simulink model "Final_Leg_Walk_V1"  (R2025b)
settings: Solver=VariableStepAuto  StartTime=0.0  StopTime=150  RelTol=0.01  AbsTol=0.01  EnableMultiTasking=on
undefined symbols (not defined in the file): X, Y, Z
libraries: sm_lib x54, nesl_utility x13
(part 3 of 3)

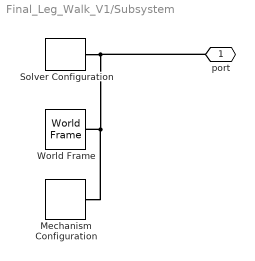
== system Final_Leg_Walk_V1/Subsystem ==
  Mechanism Configuration : sm_lib/Utilities/Mechanism Configuration  UniformGravity=Constant  GravityVector=[0 0 -9.80665]  GravityVectorUnits=m/s^2  LinearizationDelta=0.001  JointModeTransitionNonlinearIterations=2
  Solver Configuration : nesl_utility/Solver Configuration  PhysicalDomain=network_engine_domain  SubClassName=solver  LeftPortType=input  RightPortType=generic  Tones=[]  Harmonics=[]  SimulateNoise=off  Profile=off  UseLocalSampling=off  EnableSwitchedLinearOptims=on  FrequencyDomain=off  UseCCode=off  RelTol=0.001  AbsTol=1e-06  MinStep=1e-09  ToWorkspace=off  RevertToSquareIcSolve=off  NumHomotopyIterations=100  PhasorMode=off  PhasorModeNumHarmonics=1  ConsistencySolver=NEWTON_XTOL_AFTER_FTOL  IndexReductionMethod=DerivativeReplacement  DoDC=off  ResidualTolerance=1e-09  ConsistencyTolSource=GLOBAL  ConsistencyAbsTol=0.001  ConsistencyRelTol=0.001  ConsistencyTolFactor=0.001  UseLocalSolver=off  LocalSolverChoice=NE_BACKWARD_EULER_ADVANCER  ResolveIndetEquations=on  FunctionEvalNumThread=1  LocalSolverSampleTime=0.001  DoFixedCost=off  MaxNonlinIter=3  MaxModeIter=2  ComputeImpulses=off  ImpulseIterations=2  LinearAlgebra=Sparse  LinearAlgebraNumThread=0  EquationFormulation=NE_TIME_EF  DelaysMemoryBudget=1024  AutomaticFiltering=on  FilteringTimeConstant=0.001  PartitionStorageMethod=AS_NEEDED  PartitionMemoryBudget=1024  PartitionMethod=FAST  MultibodyUseLocalSolver=off  MultibodyLocalSolverChoice=ODE1  MultibodyLocalSolverSampleTime=0.001
  World Frame : sm_lib/Frames and Transforms/World Frame
  port : PMIOPort  Side=Right
  connections:
  Solver Configuration/RConn1 -- port/RConn1 -- Mechanism Configuration/RConn1 -- World Frame/RConn1

== matlab function Final_Leg_Walk_V1/RR/MATLAB Function3 ==
  data: t input; q_roll output; leg_id input; q_hip output; q_knee output
function [q_roll, q_hip, q_knee] = motion_walker_v8_extended(t, leg_id)
    % (small stepping + large backward stroke) extended to a complete
    % four-leg cycle
    % Sequence: right front (0) -> left rear (2) -> left front (1) -> right rear (3)
    
    % ================= settings =================
    T_start = 2.0;
    if t < T_start
        q_roll = 0; q_hip = 0; q_knee = 0;
        return;
    end
    t_run = t - T_start;
    
    % [1] Lean(roll) amplitude
    ang_lean = deg2rad(3); 
    
    % [2] Step amplitude (negative value moves forward)
    ang_step = deg2rad(-10); 
    
    % [3] Propulsion amplitude (positive value moves backword)
    ang_push = deg2rad(10);
    
    % [4] Leg lift amplitude
    ang_lift = deg2rad(-12); 
    
    % Period: 4 legs x (2s preparation + 2s action)=16s
    T_cycle = 16.0; 
    tau = mod(t_run, T_cycle);
    
    smooth_move = @(x) (1 - cos(x*pi))/2; 
    lift_arch   = @(x) sin(x*pi);         

    % ================= Logic =================
    q_roll = 0; q_hip = 0; q_knee = 0;
    
    % ---------------------------------------------------------
    % Phase A: Right Front, Leg 0 [0-4s]
    % ---------------------------------------------------------
    if tau < 2.0
        % [Preparation] Shift the center of mass to the left (0 -> -5)
        s = smooth_move(tau/2.0);
        q_roll = s * (-ang_lean);

        
    elseif tau < 4.0
        % [Action] Lift the right front leg
        local_t = (tau - 2.0)/2.0;
        s = smooth_move(local_t);
        q_roll = -ang_lean; % maintain left lean
        
        if leg_id == 0
            % === Main leg: right front leg ===
            q_knee = lift_arch(local_t) * ang_lift;
            q_hip = s * ang_step; 
        else
            % === Supporting legs: other legs ===
            q_knee = 0; 
            q_hip = s * ang_push; % continue backward stroke
        end

    % ---------------------------------------------------------
    % Phase B: Left Rear, Leg 2 [4-8s]
    % ---------------------------------------------------------
    elseif tau < 6.0
        % [Preparation] Shift the center of mass to the right (-5 -> +5)
        local_t = (tau - 4.0)/2.0;
        s = smooth_move(local_t);
        q_roll = -ang_lean + s * (2 * ang_lean);
        
        % Keep the leg that just stepped forward in place; the others keep
        % stroking backward
        if leg_id == 0; q_hip = ang_step; else; q_hip = ang_push; end
        
    elseif tau < 8.0
        % [Action] Lift the left rear leg
        local_t = (tau - 6.0)/2.0;
        s = smooth_move(local_t);
        q_roll = ang_lean; % Maintain right lean
        
        if leg_id == 2
            % === Main leg: left rear leg ===
            q_knee = lift_arch(local_t) * ang_lift;
            q_hip = ang_push + s * (ang_step - ang_push); % Step forward
        else
            % === Supporting legs: other legs ===
            q_knee = 0;
            % Right front leg(0) stays forward, other legs stay backward
            if leg_id == 0; q_hip = ang_step; else; q_hip = ang_push; end
        end

    % ---------------------------------------------------------
    % Phase C: Left Front, Leg 1 [8-12s]
    % ---------------------------------------------------------
    elseif tau < 10.0
         % [Preparation] Keep the center of mass on the right side (no movement)
         % Because the previous motion was the left rear leg (COM on the right),
         % and now the left front leg moves, the COM must remain on the right
        q_roll = ang_lean; 
        
        if leg_id == 0 || leg_id == 2; q_hip = ang_step; else; q_hip = ang_push; end
        
    elseif tau < 12.0
        % [Action] Lift the left front leg
        local_t = (tau - 10.0)/2.0;
        s = smooth_move(local_t);
        q_roll = ang_lean; % Maintain right lean
        
        if leg_id == 1
            % === Main leg: left front leg ===
            q_knee = lift_arch(local_t) * ang_lift;
            q_hip = ang_push + s * (ang_step - ang_push);
        else
            q_knee = 0;
            if leg_id == 0 || leg_id == 2; q_hip = ang_step; else; q_hip = ang_push; end
        end

    % ---------------------------------------------------------
    % Phase D: Right Rear, Leg 3 [12-16s]
    % ---------------------------------------------------------
    elseif tau < 14.0
        % [Preparation] Shift the center of mass from right back to the left (+5 -> -5)
        local_t = (tau - 12.0)/2.0;
        s = smooth_move(local_t);
        q_roll = ang_lean + s * (-2 * ang_lean);
        
        if leg_id == 3; q_hip = ang_push; else; q_hip = ang_step; end
        
    else
        % [Action] Lift the right rear leg
        local_t = (tau - 14.0)/2.0;
        s = smooth_move(local_t);
        q_roll = -ang_lean * (1 - s); % Left lean gradually returns to neutral
        target_pos = 0; 
        if leg_id == 3
            % === Main leg: right rear leg ===
            q_knee = lift_arch(local_t) * ang_lift;
            q_hip = ang_push + s * (target_pos - ang_push);
        else
            q_knee = 0;
            % All other legs return to neutral
            q_hip = ang_step + s * (target_pos - ang_step);
            
        end
    end
end

== matlab function Final_Leg_Walk_V1/FL/MATLAB Function3 ==
  data: t input; q_roll output; leg_id input; q_hip output; q_knee output
function [q_roll, q_hip, q_knee] = motion_walker_v8_extended(t, leg_id)
    % (small stepping + large backward stroke) extended to a complete
    % four-leg cycle
    % Sequence: right front (0) -> left rear (2) -> left front (1) -> right rear (3)
    
    % ================= settings =================
    T_start = 2.0;
    if t < T_start
        q_roll = 0; q_hip = 0; q_knee = 0;
        return;
    end
    t_run = t - T_start;
    
    % [1] Lean(roll) amplitude
    ang_lean = deg2rad(3); 
    
    % [2] Step amplitude (negative value moves forward)
    ang_step = deg2rad(-10); 
    
    % [3] Propulsion amplitude (positive value moves backword)
    ang_push = deg2rad(10);
    
    % [4] Leg lift amplitude
    ang_lift = deg2rad(-12); 
    
    % Period: 4 legs x (2s preparation + 2s action)=16s
    T_cycle = 16.0; 
    tau = mod(t_run, T_cycle);
    
    smooth_move = @(x) (1 - cos(x*pi))/2; 
    lift_arch   = @(x) sin(x*pi);         

    % ================= Logic =================
    q_roll = 0; q_hip = 0; q_knee = 0;
    
    % ---------------------------------------------------------
    % Phase A: Right Front, Leg 0 [0-4s]
    % ---------------------------------------------------------
    if tau < 2.0
        % [Preparation] Shift the center of mass to the left (0 -> -5)
        s = smooth_move(tau/2.0);
        q_roll = s * (-ang_lean);

        
    elseif tau < 4.0
        % [Action] Lift the right front leg
        local_t = (tau - 2.0)/2.0;
        s = smooth_move(local_t);
        q_roll = -ang_lean; % maintain left lean
        
        if leg_id == 0
            % === Main leg: right front leg ===
            q_knee = lift_arch(local_t) * ang_lift;
            q_hip = s * ang_step; 
        else
            % === Supporting legs: other legs ===
            q_knee = 0; 
            q_hip = s * ang_push; % continue backward stroke
        end

    % ---------------------------------------------------------
    % Phase B: Left Rear, Leg 2 [4-8s]
    % ---------------------------------------------------------
    elseif tau < 6.0
        % [Preparation] Shift the center of mass to the right (-5 -> +5)
        local_t = (tau - 4.0)/2.0;
        s = smooth_move(local_t);
        q_roll = -ang_lean + s * (2 * ang_lean);
        
        % Keep the leg that just stepped forward in place; the others keep
        % stroking backward
        if leg_id == 0; q_hip = ang_step; else; q_hip = ang_push; end
        
    elseif tau < 8.0
        % [Action] Lift the left rear leg
        local_t = (tau - 6.0)/2.0;
        s = smooth_move(local_t);
        q_roll = ang_lean; % Maintain right lean
        
        if leg_id == 2
            % === Main leg: left rear leg ===
            q_knee = lift_arch(local_t) * ang_lift;
            q_hip = ang_push + s * (ang_step - ang_push); % Step forward
        else
            % === Supporting legs: other legs ===
            q_knee = 0;
            % Right front leg(0) stays forward, other legs stay backward
            if leg_id == 0; q_hip = ang_step; else; q_hip = ang_push; end
        end

    % ---------------------------------------------------------
    % Phase C: Left Front, Leg 1 [8-12s]
    % ---------------------------------------------------------
    elseif tau < 10.0
         % [Preparation] Keep the center of mass on the right side (no movement)
         % Because the previous motion was the left rear leg (COM on the right),
         % and now the left front leg moves, the COM must remain on the right
        q_roll = ang_lean; 
        
        if leg_id == 0 || leg_id == 2; q_hip = ang_step; else; q_hip = ang_push; end
        
    elseif tau < 12.0
        % [Action] Lift the left front leg
        local_t = (tau - 10.0)/2.0;
        s = smooth_move(local_t);
        q_roll = ang_lean; % Maintain right lean
        
        if leg_id == 1
            % === Main leg: left front leg ===
            q_knee = lift_arch(local_t) * ang_lift;
            q_hip = ang_push + s * (ang_step - ang_push);
        else
            q_knee = 0;
            if leg_id == 0 || leg_id == 2; q_hip = ang_step; else; q_hip = ang_push; end
        end

    % ---------------------------------------------------------
    % Phase D: Right Rear, Leg 3 [12-16s]
    % ---------------------------------------------------------
    elseif tau < 14.0
        % [Preparation] Shift the center of mass from right back to the left (+5 -> -5)
        local_t = (tau - 12.0)/2.0;
        s = smooth_move(local_t);
        q_roll = ang_lean + s * (-2 * ang_lean);
        
        if leg_id == 3; q_hip = ang_push; else; q_hip = ang_step; end
        
    else
        % [Action] Lift the right rear leg
        local_t = (tau - 14.0)/2.0;
        s = smooth_move(local_t);
        q_roll = -ang_lean * (1 - s); % Left lean gradually returns to neutral
        target_pos = 0; 
        if leg_id == 3
            % === Main leg: right rear leg ===
            q_knee = lift_arch(local_t) * ang_lift;
            q_hip = ang_push + s * (target_pos - ang_push);
        else
            q_knee = 0;
            % All other legs return to neutral
            q_hip = ang_step + s * (target_pos - ang_step);
            
        end
    end
end

== matlab function Final_Leg_Walk_V1/FR/MATLAB Function3 ==
  data: t input; q_roll output; leg_id input; q_hip output; q_knee output
function [q_roll, q_hip, q_knee] = motion_walker_v8_extended(t, leg_id)
    % (small stepping + large backward stroke) extended to a complete
    % four-leg cycle
    % Sequence: right front (0) -> left rear (2) -> left front (1) -> right rear (3)
    
    % ================= settings =================
    T_start = 2.0;
    if t < T_start
        q_roll = 0; q_hip = 0; q_knee = 0;
        return;
    end
    t_run = t - T_start;
    
    % [1] Lean(roll) amplitude
    ang_lean = deg2rad(3); 
    
    % [2] Step amplitude (negative value moves forward)
    ang_step = deg2rad(-10); 
    
    % [3] Propulsion amplitude (positive value moves backword)
    ang_push = deg2rad(10);
    
    % [4] Leg lift amplitude
    ang_lift = deg2rad(-12); 
    
    % Period: 4 legs x (2s preparation + 2s action)=16s
    T_cycle = 16.0; 
    tau = mod(t_run, T_cycle);
    
    smooth_move = @(x) (1 - cos(x*pi))/2; 
    lift_arch   = @(x) sin(x*pi);         

    % ================= Logic =================
    q_roll = 0; q_hip = 0; q_knee = 0;
    
    % ---------------------------------------------------------
    % Phase A: Right Front, Leg 0 [0-4s]
    % ---------------------------------------------------------
    if tau < 2.0
        % [Preparation] Shift the center of mass to the left (0 -> -5)
        s = smooth_move(tau/2.0);
        q_roll = s * (-ang_lean);

        
    elseif tau < 4.0
        % [Action] Lift the right front leg
        local_t = (tau - 2.0)/2.0;
        s = smooth_move(local_t);
        q_roll = -ang_lean; % maintain left lean
        
        if leg_id == 0
            % === Main leg: right front leg ===
            q_knee = lift_arch(local_t) * ang_lift;
            q_hip = s * ang_step; 
        else
            % === Supporting legs: other legs ===
            q_knee = 0; 
            q_hip = s * ang_push; % continue backward stroke
        end

    % ---------------------------------------------------------
    % Phase B: Left Rear, Leg 2 [4-8s]
    % ---------------------------------------------------------
    elseif tau < 6.0
        % [Preparation] Shift the center of mass to the right (-5 -> +5)
        local_t = (tau - 4.0)/2.0;
        s = smooth_move(local_t);
        q_roll = -ang_lean + s * (2 * ang_lean);
        
        % Keep the leg that just stepped forward in place; the others keep
        % stroking backward
        if leg_id == 0; q_hip = ang_step; else; q_hip = ang_push; end
        
    elseif tau < 8.0
        % [Action] Lift the left rear leg
        local_t = (tau - 6.0)/2.0;
        s = smooth_move(local_t);
        q_roll = ang_lean; % Maintain right lean
        
        if leg_id == 2
            % === Main leg: left rear leg ===
            q_knee = lift_arch(local_t) * ang_lift;
            q_hip = ang_push + s * (ang_step - ang_push); % Step forward
        else
            % === Supporting legs: other legs ===
            q_knee = 0;
            % Right front leg(0) stays forward, other legs stay backward
            if leg_id == 0; q_hip = ang_step; else; q_hip = ang_push; end
        end

    % ---------------------------------------------------------
    % Phase C: Left Front, Leg 1 [8-12s]
    % ---------------------------------------------------------
    elseif tau < 10.0
         % [Preparation] Keep the center of mass on the right side (no movement)
         % Because the previous motion was the left rear leg (COM on the right),
         % and now the left front leg moves, the COM must remain on the right
        q_roll = ang_lean; 
        
        if leg_id == 0 || leg_id == 2; q_hip = ang_step; else; q_hip = ang_push; end
        
    elseif tau < 12.0
        % [Action] Lift the left front leg
        local_t = (tau - 10.0)/2.0;
        s = smooth_move(local_t);
        q_roll = ang_lean; % Maintain right lean
        
        if leg_id == 1
            % === Main leg: left front leg ===
            q_knee = lift_arch(local_t) * ang_lift;
            q_hip = ang_push + s * (ang_step - ang_push);
        else
            q_knee = 0;
            if leg_id == 0 || leg_id == 2; q_hip = ang_step; else; q_hip = ang_push; end
        end

    % ---------------------------------------------------------
    % Phase D: Right Rear, Leg 3 [12-16s]
    % ---------------------------------------------------------
    elseif tau < 14.0
        % [Preparation] Shift the center of mass from right back to the left (+5 -> -5)
        local_t = (tau - 12.0)/2.0;
        s = smooth_move(local_t);
        q_roll = ang_lean + s * (-2 * ang_lean);
        
        if leg_id == 3; q_hip = ang_push; else; q_hip = ang_step; end
        
    else
        % [Action] Lift the right rear leg
        local_t = (tau - 14.0)/2.0;
        s = smooth_move(local_t);
        q_roll = -ang_lean * (1 - s); % Left lean gradually returns to neutral
        target_pos = 0; 
        if leg_id == 3
            % === Main leg: right rear leg ===
            q_knee = lift_arch(local_t) * ang_lift;
            q_hip = ang_push + s * (target_pos - ang_push);
        else
            q_knee = 0;
            % All other legs return to neutral
            q_hip = ang_step + s * (target_pos - ang_step);
            
        end
    end
end

== matlab function Final_Leg_Walk_V1/RL/MATLAB Function2 ==
  data: t input; q_roll output; leg_id input; q_hip output; q_knee output
function [q_roll, q_hip, q_knee] = motion_walker_v8_extended(t, leg_id)
    % (small stepping + large backward stroke) extended to a complete
    % four-leg cycle
    % Sequence: right front (0) -> left rear (2) -> left front (1) -> right rear (3)
    
    % ================= settings =================
    T_start = 2.0;
    if t < T_start
        q_roll = 0; q_hip = 0; q_knee = 0;
        return;
    end
    t_run = t - T_start;
    
    % [1] Lean(roll) amplitude
    ang_lean = deg2rad(3); 
    
    % [2] Step amplitude (negative value moves forward)
    ang_step = deg2rad(-10); 
    
    % [3] Propulsion amplitude (positive value moves backword)
    ang_push = deg2rad(10);
    
    % [4] Leg lift amplitude
    ang_lift = deg2rad(-12); 
    
    % Period: 4 legs x (2s preparation + 2s action)=16s
    T_cycle = 16.0; 
    tau = mod(t_run, T_cycle);
    
    smooth_move = @(x) (1 - cos(x*pi))/2; 
    lift_arch   = @(x) sin(x*pi);         

    % ================= Logic =================
    q_roll = 0; q_hip = 0; q_knee = 0;
    
    % ---------------------------------------------------------
    % Phase A: Right Front, Leg 0 [0-4s]
    % ---------------------------------------------------------
    if tau < 2.0
        % [Preparation] Shift the center of mass to the left (0 -> -5)
        s = smooth_move(tau/2.0);
        q_roll = s * (-ang_lean);

        
    elseif tau < 4.0
        % [Action] Lift the right front leg
        local_t = (tau - 2.0)/2.0;
        s = smooth_move(local_t);
        q_roll = -ang_lean; % maintain left lean
        
        if leg_id == 0
            % === Main leg: right front leg ===
            q_knee = lift_arch(local_t) * ang_lift;
            q_hip = s * ang_step; 
        else
            % === Supporting legs: other legs ===
            q_knee = 0; 
            q_hip = s * ang_push; % continue backward stroke
        end

    % ---------------------------------------------------------
    % Phase B: Left Rear, Leg 2 [4-8s]
    % ---------------------------------------------------------
    elseif tau < 6.0
        % [Preparation] Shift the center of mass to the right (-5 -> +5)
        local_t = (tau - 4.0)/2.0;
        s = smooth_move(local_t);
        q_roll = -ang_lean + s * (2 * ang_lean);
        
        % Keep the leg that just stepped forward in place; the others keep
        % stroking backward
        if leg_id == 0; q_hip = ang_step; else; q_hip = ang_push; end
        
    elseif tau < 8.0
        % [Action] Lift the left rear leg
        local_t = (tau - 6.0)/2.0;
        s = smooth_move(local_t);
        q_roll = ang_lean; % Maintain right lean
        
        if leg_id == 2
            % === Main leg: left rear leg ===
            q_knee = lift_arch(local_t) * ang_lift;
            q_hip = ang_push + s * (ang_step - ang_push); % Step forward
        else
            % === Supporting legs: other legs ===
            q_knee = 0;
            % Right front leg(0) stays forward, other legs stay backward
            if leg_id == 0; q_hip = ang_step; else; q_hip = ang_push; end
        end

    % ---------------------------------------------------------
    % Phase C: Left Front, Leg 1 [8-12s]
    % ---------------------------------------------------------
    elseif tau < 10.0
         % [Preparation] Keep the center of mass on the right side (no movement)
         % Because the previous motion was the left rear leg (COM on the right),
         % and now the left front leg moves, the COM must remain on the right
        q_roll = ang_lean; 
        
        if leg_id == 0 || leg_id == 2; q_hip = ang_step; else; q_hip = ang_push; end
        
    elseif tau < 12.0
        % [Action] Lift the left front leg
        local_t = (tau - 10.0)/2.0;
        s = smooth_move(local_t);
        q_roll = ang_lean; % Maintain right lean
        
        if leg_id == 1
            % === Main leg: left front leg ===
            q_knee = lift_arch(local_t) * ang_lift;
            q_hip = ang_push + s * (ang_step - ang_push);
        else
            q_knee = 0;
            if leg_id == 0 || leg_id == 2; q_hip = ang_step; else; q_hip = ang_push; end
        end

    % ---------------------------------------------------------
    % Phase D: Right Rear, Leg 3 [12-16s]
    % ---------------------------------------------------------
    elseif tau < 14.0
        % [Preparation] Shift the center of mass from right back to the left (+5 -> -5)
        local_t = (tau - 12.0)/2.0;
        s = smooth_move(local_t);
        q_roll = ang_lean + s * (-2 * ang_lean);
        
        if leg_id == 3; q_hip = ang_push; else; q_hip = ang_step; end
        
    else
        % [Action] Lift the right rear leg
        local_t = (tau - 14.0)/2.0;
        s = smooth_move(local_t);
        q_roll = -ang_lean * (1 - s); % Left lean gradually returns to neutral
        target_pos = 0; 
        if leg_id == 3
            % === Main leg: right rear leg ===
            q_knee = lift_arch(local_t) * ang_lift;
            q_hip = ang_push + s * (target_pos - ang_push);
        else
            q_knee = 0;
            % All other legs return to neutral
            q_hip = ang_step + s * (target_pos - ang_step);
            
        end
    end
end
